simulink model "atrias_boom_nmSt_kinSw_v3"  (R2015a)
settings: Solver=ode23t  StartTime=0.0  StopTime=t_end  FixedStep=0.001  MaxStep=1e-3  RelTol=1e-3
InitFcn:
  | addpath('../common/')
  | colors
StartFcn:
  | tic
StopFcn:
  | %stopscript
values from neighbouring files (symbols this model uses):
  dt_a_dTrunk_boom = 5    [main_1_nmSt_kinSw.m]    (also in main_2_nmSt_kinSw_v2.m; main_3_nmSt_kinSw_v3.m; main_4_nmSt_kinSw_v4.m)
  dt_fade_boomCtrl = 2    [main_1_nmSt_kinSw.m]    (also in main_2_nmSt_kinSw_v2.m; main_3_nmSt_kinSw_v3.m; main_4_nmSt_kinSw_v4.m)
  initial_boom_yaw = 15*pi/180    (= 0.261799387799)    [main_2_nmSt_kinSw_v2.m]    (also in main_3_nmSt_kinSw_v3.m; main_4_nmSt_kinSw_v4.m)
  kd_boom_roll_Ctrl = 0    [main_1_nmSt_kinSw - Copy.m]    (also in main_1_nmSt_kinSw.m; main_2_nmSt_kinSw_v2.m; main_3_nmSt_kinSw_v3.m; main_4_nmSt_kinSw_v4.m)
  kd_boom_yaw_Ctrl = 0.1*kp_boom_yaw_Ctrl    (= 100000000)    [main_1_nmSt_kinSw - Copy.m]    (also in main_1_nmSt_kinSw.m = 1000000000; main_2_nmSt_kinSw_v2.m = 10000000; main_3_nmSt_kinSw_v3.m = 10000000; main_4_nmSt_kinSw_v4.m = 10000000)
  kd_motor = 0.90*2*sqrt(3.75*kp_motor)    [main_1_nmSt_kinSw - Copy.m]
  kinSw_alpha_start = 100*pi/180    (= 1.74532925199)    [main_1_nmSt_kinSw - Copy.m]    (also in main_1_nmSt_kinSw.m = 1.91986217719; main_2_nmSt_kinSw_v2.m = 1.83259571459; main_3_nmSt_kinSw_v3.m = 1.83259571459; main_4_nmSt_kinSw_v4.m = 1.83259571459)
  kinSw_alpha_tgt = 80*pi/180    (= 1.3962634016)    [main_1_nmSt_kinSw - Copy.m]    (also in main_1_nmSt_kinSw.m = 1.2217304764; main_2_nmSt_kinSw_v2.m = 1.2217304764; main_3_nmSt_kinSw_v3.m = 1.2217304764; main_4_nmSt_kinSw_v4.m = 1.2217304764)
  kinSw_t_start = 1.5    [main_1_nmSt_kinSw - Copy.m]    (also in main_1_nmSt_kinSw.m; main_2_nmSt_kinSw_v2.m = 0.5; main_3_nmSt_kinSw_v3.m = 0.5; main_4_nmSt_kinSw_v4.m = 0.5)
  kp_boom_roll_Ctrl = 0    [main_1_nmSt_kinSw - Copy.m]    (also in main_1_nmSt_kinSw.m; main_2_nmSt_kinSw_v2.m; main_3_nmSt_kinSw_v3.m; main_4_nmSt_kinSw_v4.m)
  kp_boom_yaw_Ctrl = 1e9    (= 1000000000)    [main_1_nmSt_kinSw - Copy.m]    (also in main_1_nmSt_kinSw.m = 10000000000; main_2_nmSt_kinSw_v2.m = 100000000; main_3_nmSt_kinSw_v3.m = 100000000; main_4_nmSt_kinSw_v4.m = 100000000)
  kp_motor = 3000    [main_1_nmSt_kinSw - Copy.m]
  max_back_bar_angle = 262.4*pi/180    (= 4.57974395723)    [main_1_nmSt_kinSw - Copy.m]
  max_front_bar_angle = 194.8*pi/180    (= 3.39990138288)    [main_1_nmSt_kinSw - Copy.m]
  min_back_bar_angle = 165.0*pi/180    (= 2.87979326579)    [main_1_nmSt_kinSw - Copy.m]
  min_front_bar_angle = 98.0*pi/180    (= 1.71042266695)    [main_1_nmSt_kinSw - Copy.m]
  poser_LLegAlp = (initial_l_leg_angle -pi/2)*180/pi    (= 105)    [main_2_nmSt_kinSw_v2.m]    (also in main_3_nmSt_kinSw_v3.m; main_4_nmSt_kinSw_v4.m)
  poser_LLegLen = initial_l_leg_length    (= 0.88)    [main_2_nmSt_kinSw_v2.m]    (also in main_3_nmSt_kinSw_v3.m; main_4_nmSt_kinSw_v4.m)
  poser_RLegAlp = (initial_r_leg_angle -pi/2)*180/pi    (= 75)    [main_2_nmSt_kinSw_v2.m]    (also in main_3_nmSt_kinSw_v3.m; main_4_nmSt_kinSw_v4.m)
  poser_RLegLen = initial_r_leg_length    (= 0.9)    [main_2_nmSt_kinSw_v2.m]    (also in main_3_nmSt_kinSw_v3.m; main_4_nmSt_kinSw_v4.m)
  tEnd_boomCtrl = t_end    (= 20)    [main_1_nmSt_kinSw - Copy.m]    (also in main_1_nmSt_kinSw.m = 3; main_2_nmSt_kinSw_v2.m = 7.5; main_3_nmSt_kinSw_v3.m = 7.5; main_4_nmSt_kinSw_v4.m = 7.5)
  tStart_boomCtrl = 1    [main_1_nmSt_kinSw - Copy.m]    (also in main_1_nmSt_kinSw.m = 0; main_2_nmSt_kinSw_v2.m = 0.5; main_3_nmSt_kinSw_v3.m = 0.5; main_4_nmSt_kinSw_v4.m = 0.5)
  tune_kinSw_alpha_start = kinSw_alpha_start*180/pi    (= 105)    [main_2_nmSt_kinSw_v2.m]    (also in main_3_nmSt_kinSw_v3.m; main_4_nmSt_kinSw_v4.m)
  tune_kinSw_alpha_tgt = kinSw_alpha_tgt*180/pi    (= 70)    [main_2_nmSt_kinSw_v2.m]    (also in main_3_nmSt_kinSw_v3.m; main_4_nmSt_kinSw_v4.m)
  tune_kinSw_len_min = kinSw_lclr    (= 0.7)    [main_2_nmSt_kinSw_v2.m]    (also in main_3_nmSt_kinSw_v3.m = 0.6)
  tune_kinSw_len_tgt = kinSw_len_tgt    (= 0.9)    [main_2_nmSt_kinSw_v2.m]    (also in main_3_nmSt_kinSw_v3.m)
  tune_M1_G = St_FGain_VAS*FmaxVAS    [main_2_nmSt_kinSw_v2.m]    (also in main_3_nmSt_kinSw_v3.m; main_4_nmSt_kinSw_v4.m)
  tune_M3_0 = CtrlPar_theta0*180/pi    [main_2_nmSt_kinSw_v2.m]    (also in main_3_nmSt_kinSw_v3.m; main_4_nmSt_kinSw_v4.m)
  tune_M3_D = St_GainDTh_HFL    [main_2_nmSt_kinSw_v2.m]    (also in main_3_nmSt_kinSw_v3.m; main_4_nmSt_kinSw_v4.m)
  tune_M3_P = St_GainTh_HFL    [main_2_nmSt_kinSw_v2.m]    (also in main_3_nmSt_kinSw_v3.m; main_4_nmSt_kinSw_v4.m)
  tune_M4_G = 1    [main_3_nmSt_kinSw_v3.m]    (also in main_4_nmSt_kinSw_v4.m)
  v_dTrunk_boom = 1.3    [main_1_nmSt_kinSw.m]    (also in main_2_nmSt_kinSw_v2.m; main_3_nmSt_kinSw_v3.m; main_4_nmSt_kinSw_v4.m)
undefined symbols (not defined in the file or in its folder): A1_notch_f1, A2_notch_f1, A_lpf_dtau, A_lpf_velocity, ankle_stiffness, B1_lpf_dtau, B1_lpf_velocity, B1_notch_f1, B2_lpf_dtau, B2_lpf_velocity, B2_notch_f1, b_hmotor, b_leg_spring, b_rotor, base_color_d, boom_color_d, boom_mount_to_center_diagonal, breakaway_friction, c_jointstop, contactThr, coulomb_friction, d_com, delta_phi_max, delta_phi_max_buffer, delta_phi_max_dropoff, delta_phi_min, fblink_color_d, floor_color_d, FmaxBFSH, FmaxGLU, FmaxHAM, FmaxHFL, FmaxRF, FmaxVAS, foot_color_d, FPCtrlPar, friction_linear_zone, g, gain_nodes_sea_torque, HIP_MTR_MAX_CONT_TORQUE, HIP_MTR_MAX_TORQUE, hshaft_color_d, initial_boom_pitch, initial_boom_roll, initial_hip_roll, initial_winch_angle, j_motor, k_gn, k_gt, k_leg_spring, K_notch_f1, k_phi, k_sea, Kb_leg, kd_lateral, kd_shin_max, kd_shin_min, kd_splay_max, kd_splay_min, kd_thigh_max ... (+186)
libraries: sm_lib x210, nesl_utility x140, simulink x65, simulink_extras x32, fl_lib x16, mblibv1 x2, commnoisgen2 x1
(part 10 of 17)

== system atrias_boom_nmSt_kinSw_v3/Mechanical System Layer/R Leg/Mechanical Limits/Shin Max Collision Model ==
  note: Mechanical Limits Model
  phi [rad] : Inport
  vphi [rad/s] : Inport  Port=2
  Contact! : EnablePort  StatesWhenEnabling=reset
  Gain3 : Gain  Gain=k_phi
  Gain4 : Gain  Gain=1/v_phi_max
  Mux1 : Mux  Inputs=2
  Reaction Force : Fcn  Expr="- u(1)  *  (1-u(2)) * (u(2)<1)"
  tau_interaction[Nm] : Outport  OutputWhenDisabled=reset  InitialOutput=0
      settings: AttributesFormatString=initial = '%<InitialOutput>'\nwhen disabled = '%<OutputWhenDisabled>'
  wires:
  Gain4/1 -> Mux1/2
  Gain3/1 -> Mux1/1
  Mux1/1 -> Reaction Force/1
  vphi [rad/s]/1 -> Gain4/1
  phi [rad]/1 -> Gain3/1
  Reaction Force/1 -> tau_interaction[Nm]/1

== system atrias_boom_nmSt_kinSw_v3/Mechanical System Layer/R Leg/Mechanical Limits/Shin Min Collision Model ==
  note: Mechanical Limits Model
  phi [rad] : Inport
  vphi [rad/s] : Inport  Port=2
  Contact! : EnablePort  StatesWhenEnabling=reset
  Gain3 : Gain  Gain=k_phi
  Gain4 : Gain  Gain=1/v_phi_max
  Mux1 : Mux  Inputs=2
  Reaction Force : Fcn  Expr="- u(1)  *  (1-u(2)) * (u(2)<1)"
  tau_interaction[Nm] : Outport  OutputWhenDisabled=reset  InitialOutput=0
      settings: AttributesFormatString=initial = '%<InitialOutput>'\nwhen disabled = '%<OutputWhenDisabled>'
  wires:
  Gain4/1 -> Mux1/2
  Gain3/1 -> Mux1/1
  Mux1/1 -> Reaction Force/1
  vphi [rad/s]/1 -> Gain4/1
  phi [rad]/1 -> Gain3/1
  Reaction Force/1 -> tau_interaction[Nm]/1

== system atrias_boom_nmSt_kinSw_v3/Mechanical System Layer/R Leg/Mechanical Limits/Thigh Max Collision Model ==
  note: Mechanical Limits Model
  phi [rad] : Inport
  vphi [rad/s] : Inport  Port=2
  Contact! : EnablePort  StatesWhenEnabling=reset
  Gain3 : Gain  Gain=k_phi
  Gain4 : Gain  Gain=1/v_phi_max
  Mux1 : Mux  Inputs=2
  Reaction Force : Fcn  Expr="- u(1)  *  (1-u(2)) * (u(2)<1)"
  tau_interaction[Nm] : Outport  OutputWhenDisabled=reset  InitialOutput=0
      settings: AttributesFormatString=initial = '%<InitialOutput>'\nwhen disabled = '%<OutputWhenDisabled>'
  wires:
  Gain4/1 -> Mux1/2
  Gain3/1 -> Mux1/1
  Mux1/1 -> Reaction Force/1
  vphi [rad/s]/1 -> Gain4/1
  phi [rad]/1 -> Gain3/1
  Reaction Force/1 -> tau_interaction[Nm]/1

== system atrias_boom_nmSt_kinSw_v3/Mechanical System Layer/R Leg/Mechanical Limits/Thigh Min Collision Model ==
  note: Mechanical Limits Model
  phi [rad] : Inport
  vphi [rad/s] : Inport  Port=2
  Contact! : EnablePort  StatesWhenEnabling=reset
  Gain3 : Gain  Gain=k_phi
  Gain4 : Gain  Gain=1/v_phi_max
  Mux1 : Mux  Inputs=2
  Reaction Force : Fcn  Expr="- u(1)  *  (1-u(2)) * (u(2)<1)"
  tau_interaction[Nm] : Outport  OutputWhenDisabled=reset  InitialOutput=0
      settings: AttributesFormatString=initial = '%<InitialOutput>'\nwhen disabled = '%<OutputWhenDisabled>'
  wires:
  Reaction Force/1 -> tau_interaction[Nm]/1
  phi [rad]/1 -> Gain3/1
  vphi [rad/s]/1 -> Gain4/1
  Mux1/1 -> Reaction Force/1
  Gain3/1 -> Mux1/1
  Gain4/1 -> Mux1/2

== system atrias_boom_nmSt_kinSw_v3/Mechanical System Layer/R Leg/Mechanical Limits/Thigh-Shin Collision Model ==
  note: Mechanical Limits Model
  delta_phi [rad] : Inport
  vphi [rad/s] : Inport  Port=2
  Contact! : EnablePort  StatesWhenEnabling=reset
  Gain3 : Gain  Gain=k_phi
  Gain4 : Gain  Gain=1/v_phi_max
  Mux1 : Mux  Inputs=2
  Reaction Force : Fcn  Expr="- u(1)  *  (1-u(2)) * (u(2)<1)"
  tau_interaction[Nm] : Outport  OutputWhenDisabled=reset  InitialOutput=0
      settings: AttributesFormatString=initial = '%<InitialOutput>'\nwhen disabled = '%<OutputWhenDisabled>'
  wires:
  Reaction Force/1 -> tau_interaction[Nm]/1
  delta_phi [rad]/1 -> Gain3/1
  vphi [rad/s]/1 -> Gain4/1
  Mux1/1 -> Reaction Force/1
  Gain3/1 -> Mux1/1
  Gain4/1 -> Mux1/2

== system atrias_boom_nmSt_kinSw_v3/Mechanical System Layer/R Leg/Mechanical Limits/Thigh-Shin Collision Model1 ==
  note: Mechanical Limits Model
  delta_phi [rad] : Inport
  vphi [rad/s] : Inport  Port=2
  Contact! : EnablePort  StatesWhenEnabling=reset
  Gain3 : Gain  Gain=k_phi
  Gain4 : Gain  Gain=1/v_phi_max
  Mux1 : Mux  Inputs=2
  Reaction Force : Fcn  Expr="- u(1)  *  (1-u(2)) * (u(2)<1)"
  tau_interaction[Nm] : Outport  OutputWhenDisabled=reset  InitialOutput=0
      settings: AttributesFormatString=initial = '%<InitialOutput>'\nwhen disabled = '%<OutputWhenDisabled>'
  wires:
  Reaction Force/1 -> tau_interaction[Nm]/1
  delta_phi [rad]/1 -> Gain3/1
  vphi [rad/s]/1 -> Gain4/1
  Mux1/1 -> Reaction Force/1
  Gain3/1 -> Mux1/1
  Gain4/1 -> Mux1/2

== system atrias_boom_nmSt_kinSw_v3/Mechanical System Layer/R Leg/Shin/Frame Data ==
  Kinematic Data : ToWorkspace  VariableName=r_shin_out  SampleTime=output_sample_time
      settings: Save2DSignal=2-D array (concatenate along first dimension)
  Mux : Mux
  PS-Simulink Converter{,1..3} (4 alike) : nesl_utility/PS-Simulink Converter  PhysicalDomain=network_engine_domain  SubClassName=ps_output  LeftPortType=input  RightPortType=output  PseudoPeriodic=off  Frequencies=[]  Unit=1  AffineConversion=off
  Transform Sensor : sm_lib/Frames and Transforms/Transform Sensor  MeasurementFrame=World  SenseAngle=off  SenseAxis=off  SenseAngle1=off  SenseAngle2=off  SenseAngle3=off  SenseQ=on  SenseR=off  SenseOmegaX=off  SenseOmegaY=off  SenseOmegaZ=off  SenseOmega1=off  SenseOmega2=off  SenseOmega3=off  SenseQDot=off  SenseRDot=off  SenseAlphaX=off  SenseAlphaY=off  SenseAlphaZ=off  SenseAlpha1=off  SenseAlpha2=off  SenseAlpha3=off  SenseQDDot=off  SenseRDDot=off  SenseX=on  SenseY=on  SenseZ=on  SenseRad=off  SenseAzim=off  SenseDist=off  SenseInc=off  SenseXDot=off  SenseYDot=off  SenseZDot=off  SenseRadDot=off  SenseAzimDot=off  SenseDistDot=off  SenseIncDot=off  SenseXDDot=off  SenseYDDot=off  SenseZDDot=off  SenseRadDDot=off  SenseAzimDDot=off  SenseDistDDot=off  SenseIncDDot=off  BlockFunction=simmechanics.library.frames_transforms.transform_sensor
  World Frame : sm_lib/Frames and Transforms/World Frame  BlockFunction=simmechanics.library.frames_transforms.world_frame
  Frame : PMIOPort  Port=1  Side=Left
  wires:
  Mux/1 -> Kinematic Data/1
  PS-Simulink Converter/1 -> Mux/1
  PS-Simulink Converter1/1 -> Mux/2
  PS-Simulink Converter2/1 -> Mux/3
  PS-Simulink Converter3/1 -> Mux/4
  connections:
  PS-Simulink Converter3/LConn1 -- Transform Sensor/RConn5
  PS-Simulink Converter2/LConn1 -- Transform Sensor/RConn4
  PS-Simulink Converter1/LConn1 -- Transform Sensor/RConn3
  PS-Simulink Converter/LConn1 -- Transform Sensor/RConn2
  Transform Sensor/RConn1 -- Frame/RConn1
  Transform Sensor/LConn1 -- World Frame/RConn1

== system atrias_boom_nmSt_kinSw_v3/Mechanical System Layer/R Leg/Shin SEA/Motor Controller ==
  Desired Current [A] : Inport
  Measured Current [A] : Inport  Port=2
  Speed [rad/s] : Inport  Port=3
  Ke : Gain  Gain=Kb_leg
  PI Controller : simulink/Continuous/PID Controller  Controller=PI  TimeDomain=Continuous-time  SampleTime=-1  IntegratorMethod=Trapezoidal  FilterMethod=Forward Euler  Form=Parallel  UseFilter=on  ControllerParametersSource=internal  P=0.57  I=0.016  D=0.016  N=10  InitialConditionSource=internal  InitialConditionForIntegrator=0  InitialConditionForFilter=0  ExternalReset=none  ZeroCross=off  LimitOutput=off  UpperSaturationLimit=inf  LowerSaturationLimit=-inf  LinearizeAsGain=on  AntiWindupMode=none  Kb=1  TrackingMode=off  Kt=1  PParamMin=[]  PParamMax=[]  IParamMin=[]  IParamMax=[]  DParamMin=[]  DParamMax=[]  NParamMin=[]  NParamMax=[]  KbParamMin=[]  KbParamMax=[]  KtParamMin=[]  KtParamMax=[]  POutMin=[]  POutMax=[]  IOutMin=[]  IOutMax=[]  DOutMin=[]  DOutMax=[]  NOutMin=[]  NOutMax=[]  KbOutMin=[]  KbOutMax=[]  KtOutMin=[]  KtOutMax=[]  IntegratorOutMin=[]  IntegratorOutMax=[]  FilterOutMin=[]  FilterOutMax=[]  SumOutMin=[]  SumOutMax=[]  SumI1OutMin=[]  SumI1OutMax=[]  SumI2OutMin=[]  SumI2OutMax=[]  SumI3OutMin=[]  SumI3OutMax=[]  SumDOutMin=[]  SumDOutMax=[]  SaturationOutMin=[]  SaturationOutMax=[]  IntegratorContinuousStateAttributes=''  IntegratorStateMustResolveToSignalObject=off  IntegratorRTWStateStorageClass=Auto  FilterContinuousStateAttributes=''  FilterStateMustResolveToSignalObject=off  FilterRTWStateStorageClass=Auto  DifferentiatorICPrevScaledInput=0  DifferentiatorOutMin=[]  DifferentiatorOutMax=[]
  Resistance : Gain  Gain=R_leg
  Sum : Sum  Inputs=|+-
  Sum1 : Sum  Inputs=|++
  Sum2 : Sum  Inputs=+|+
  Voltage [V] : Outport
  wires:
  Desired Current [A]/1 -> Sum/1
  Measured Current [A]/1 -> Resistance/1, Sum/2
  Sum/1 -> PI Controller/1
  PI Controller/1 -> Sum1/1
  Speed [rad/s]/1 -> Ke/1
  Sum2/1 -> Sum1/2
  Resistance/1 -> Sum2/1
  Ke/1 -> Sum2/2
  Sum1/1 -> Voltage [V]/1

== system atrias_boom_nmSt_kinSw_v3/Mechanical System Layer/R Leg/Shin SEA/Motor Electromagnetism ==
  Voltage [V] : Inport
  Speed [rad/s] : Inport  Port=2
  Add : Sum  Inputs=-+-
  Inductance : Gain  Gain=1/L_leg
  Integrator : Integrator  ZeroCross=off
  Ke : Gain  Gain=Kb_leg
  Resistance : Gain  Gain=R_leg
  Torque Limiter (outside) 1 : Saturate  UpperLimit=max_voltage_leg  LowerLimit=-max_voltage_leg  ZeroCross=off
      settings: AttributesFormatString=Hi: %<UpperLimit>\nLo: %<LowerLimit>
  Torque Limiter (outside) 2 : Saturate  UpperLimit=max_current_leg  LowerLimit=-max_current_leg  ZeroCross=off
      settings: AttributesFormatString=Hi: %<UpperLimit>\nLo: %<LowerLimit>
  Current [A] : Outport
  wires:
  Integrator/1 -> Torque Limiter (outside) 2/1  "I"
  Inductance/1 -> Integrator/1  "d/dt(I)"
  Speed [rad/s]/1 -> Ke/1  "d/dt(theta)"
  Add/1 -> Inductance/1
  Resistance/1 -> Add/1
  Ke/1 -> Add/3
  Voltage [V]/1 -> Torque Limiter (outside) 1/1
  Torque Limiter (outside) 1/1 -> Add/2
  Torque Limiter (outside) 2/1 -> Resistance/1, Current [A]/1

== system atrias_boom_nmSt_kinSw_v3/Mechanical System Layer/R Leg/Shin SEA/Rotor and Gearing ==
  Rotor Torque [Nm] : Inport
  Spring Torque [Nm] : Inport  Port=2
  Aligned Gear Constraint : sm_lib/Gears and Couplings/Gears/Common Gear Constraint  GearType=External  SpecificationType=CenterDistanceRatio  CenterDistance=(r_rotor+r_virtual_gear)/2  CenterDistanceUnits=m  GearRatio=1  BaseGearRadius=1  BaseGearRadiusUnits=m  FollGearRadius=1  FollGearRadiusUnits=m  AssemblyGearRotation=Free  BlockFunction=simmechanics.library.gears_couplings_drives.gears.common_gear
  External Force and Torque : sm_lib/Forces and Torques/External Force and Torque  ForceResolutionFrame=AttachedFrame  EnableForceX=off  EnableForceY=off  EnableForceZ=off  EnableForce=off  TorqueResolutionFrame=AttachedFrame  EnableTorqueX=off  EnableTorqueY=off  EnableTorqueZ=on  EnableTorque=off  BlockFunction=simmechanics.library.forces_torques.external_force_torque
  Gear Offset : sm_lib/Frames and Transforms/Rigid Transform  TranslationMethod=Cartesian  TranslationLengthUnit=m  TranslationStandardAxis=+Z  TranslationStandardOffset=0  TranslationCartesianOffset=[(r_rotor+r_virtual_gear) 0 0]  TranslationROffset=0  TranslationROffsetUnits=m  TranslationZOffset=0  TranslationZOffsetUnits=m  TranslationThetaOffset=0  TranslationThetaOffsetUnits=deg  RotationMethod=None  RotationAngleUnits=deg  RotationStandardAxis=+Z  RotationAngle=0  RotationArbitraryAxis=[0 0 1]  FollAlignAxisA=+X  BaseAlignAxisA=+Y  FollAlignAxisB=+Y  BaseAlignAxisB=+Z  RotationMatrix=[1 0 0; 0 1 0; 0 0 1]  BlockFunction=simmechanics.library.frames_transforms.rigid_transform
  Idler Gear : sm_lib/Body Elements/Solid  InertiaType=Custom  Mass=m_virtual_gear  MassUnits=kg  CenterOfMass=[0 0 0]  CenterOfMassUnits=m  MomentsOfInertia=i_virtual_gear  MomentsOfInertiaUnits=kg*m^2  ProductsOfInertia=[0 0 0]  ProductsOfInertiaUnits=kg*m^2  DensityBased=on  Density=1000  DensityUnits=kg/(m^3)  GraphicType=None  MarkerShape=Sphere  MarkerSize=10  MarkerSizeUnits=m  GraphicVisPropType=SimpleVisualProperties  GraphicDiffuseColor=[1.0 0.2 0.2]  GraphicSpecularColor=[0.5 0.5 0.5 1.0]  GraphicAmbientColor=[0.15 0.15 0.15 1.0]  GraphicEmissiveColor=[0.0 0.0 0.0 1.0]  GraphicShininess=75  GraphicOpacity=1.0  GeometryShape=Cylinder  RectangleSize=[1 1]  RectangleSizeUnits=m  BrickDimensions=[1 1 1]  BrickDimensionUnits=m  CylinderRadius=r_virtual_gear  CylinderRadiusUnits=m  CylinderLength=0.01  CylinderLengthUnits=m  SphereRadius=1  SphereRadiusUnits=m  EllipsoidRadii=[1 1 1]  EllipsoidRadiiUnits=m  ExtrusionCrossSection=[1 1; -1 1; -1 -1; 1 -1]  ExtrusionCrossSectionUnits=m  ExtrusionLength=.2  ExtrusionLengthUnits=m  PolygonNumSides=3  PolygonOuterRadius=.3  PolygonOuterRadiusUnits=m  ExtGeomFileType=STL  ExtGeomFileUnits=m  RevolutionCrossSection=[1 1; 1 -1; 2 -1; 2 1]  RevolutionCrossSectionUnits=m  RevolutionExtent=Full  RevolutionAngle=180  RevolutionAngleUnits=deg  BlockFunction=simmechanics.library.body_elements.solid
  Idler Gear Constraint : sm_lib/Gears and Couplings/Gears/Common Gear Constraint  GearType=External  SpecificationType=CenterDistanceRatio  CenterDistance=(r_rotor+r_virtual_gear)/2  CenterDistanceUnits=m  GearRatio=1.0  BaseGearRadius=r_rotor  BaseGearRadiusUnits=m  FollGearRadius=r_virtual_gear  FollGearRadiusUnits=m  AssemblyGearRotation=Free  BlockFunction=simmechanics.library.gears_couplings_drives.gears.common_gear
  Idler Offset : sm_lib/Frames and Transforms/Rigid Transform  TranslationMethod=Cartesian  TranslationLengthUnit=m  TranslationStandardAxis=+Z  TranslationStandardOffset=0  TranslationCartesianOffset=[(r_rotor+r_virtual_gear)/2 0 0]  TranslationROffset=0  TranslationROffsetUnits=m  TranslationZOffset=0  TranslationZOffsetUnits=m  TranslationThetaOffset=0  TranslationThetaOffsetUnits=deg  RotationMethod=None  RotationAngleUnits=deg  RotationStandardAxis=+Z  RotationAngle=0  RotationArbitraryAxis=[0 0 1]  FollAlignAxisA=+X  BaseAlignAxisA=+Y  FollAlignAxisB=+Y  BaseAlignAxisB=+Z  RotationMatrix=[1 0 0; 0 1 0; 0 0 1]  BlockFunction=simmechanics.library.frames_transforms.rigid_transform
  Mechanical Rotational Reference : fl_lib/Mechanical/Rotational Elements/Mechanical Rotational Reference
  Opposite : Gain  Gain=-1
  Output Gear Joint : sm_lib/Joints/Revolute Joint  SenseConstraintForce=off  SenseConstraintForceX=off  SenseConstraintForceY=off  SenseConstraintForceZ=off  SenseConstraintTorque=off  SenseConstraintTorqueX=off  SenseConstraintTorqueY=off  SenseConstraintTorqueZ=off  SenseTotalForce=off  SenseTotalForceX=off  SenseTotalForceY=off  SenseTotalForceZ=off  SenseTotalTorque=off  SenseTotalTorqueX=off  SenseTotalTorqueY=off  SenseTotalTorqueZ=off  CompositeWrenchDir=FollowerOnBase  CompositeWrenchFrame=BaseFrame  EquilibriumPosition=0  EquilibriumPositionUnits=deg  SpringStiffness=0  SpringStiffnessUnits=N*m/deg  DampingCoefficient=0  DampingCoefficientUnits=N*m/(deg/s)  TorqueActuationMode=NoTorque  MotionActuationMode=ComputedMotion  SensePosition=on  SenseVelocity=on  SenseAcceleration=off  SenseTorqueForce=off  PositionTargetSpecify=off  PositionTargetPriority=High  PositionTargetValue=0  PositionTargetValueUnits=deg  VelocityTargetSpecify=off  VelocityTargetPriority=High  VelocityTargetValue=0  VelocityTargetValueUnits=deg/s  BlockFunction=simmechanics.library.joints.revolute_joint
  Output Gear : sm_lib/Body Elements/Solid  InertiaType=Custom  Mass=m_output_gear  MassUnits=kg  CenterOfMass=[0 0 0]  CenterOfMassUnits=m  MomentsOfInertia=i_output_gear  MomentsOfInertiaUnits=kg*m^2  ProductsOfInertia=[0 0 0]  ProductsOfInertiaUnits=kg*m^2  DensityBased=on  Density=1000  DensityUnits=kg/(m^3)  GraphicType=None  MarkerShape=Sphere  MarkerSize=10  MarkerSizeUnits=m  GraphicVisPropType=SimpleVisualProperties  GraphicDiffuseColor=[1.0 0.2 0.0]  GraphicSpecularColor=[0.5 0.5 0.5 1.0]  GraphicAmbientColor=[0.15 0.15 0.15 1.0]  GraphicEmissiveColor=[0.0 0.0 0.0 1.0]  GraphicShininess=75  GraphicOpacity=1.0  GeometryShape=Cylinder  RectangleSize=[1 1]  RectangleSizeUnits=m  BrickDimensions=[1 1 1]  BrickDimensionUnits=m  CylinderRadius=0.03  CylinderRadiusUnits=m  CylinderLength=0.01  CylinderLengthUnits=m  SphereRadius=1  SphereRadiusUnits=m  EllipsoidRadii=[1 1 1]  EllipsoidRadiiUnits=m  ExtrusionCrossSection=[1 1; -1 1; -1 -1; 1 -1]  ExtrusionCrossSectionUnits=m  ExtrusionLength=1  ExtrusionLengthUnits=m  PolygonNumSides=3  PolygonOuterRadius=1  PolygonOuterRadiusUnits=m  ExtGeomFileType=STL  ExtGeomFileUnits=m  RevolutionCrossSection=[1 1; 1 -1; 2 -1; 2 1]  RevolutionCrossSectionUnits=m  RevolutionExtent=Full  RevolutionAngle=180  RevolutionAngleUnits=deg  BlockFunction=simmechanics.library.body_elements.solid
  PS-Simulink Converter{,1..3} (4 alike) : nesl_utility/PS-Simulink Converter  PhysicalDomain=network_engine_domain  SubClassName=ps_output  LeftPortType=input  RightPortType=output  PseudoPeriodic=off  Frequencies=[]  Unit=1  AffineConversion=off
  Rotational Simscape Intf : Subsystem
  Rotational Friction : fl_lib/Mechanical/Rotational Elements/Rotational Friction  brkwy_trq=breakaway_friction(1)/N N*m  Col_trq=coulomb_friction(1)/N N*m  visc_coef=viscous_friction(1)/N N*m/(rad/s)  trans_coef=10 s/rad  vel_thr=friction_linear_zone(1)*N rad/s  w_specify=off  w_priority=High  w=0 rad/s  t_specify=off  t_priority=High  t=0 N*m
  Rotor + Base Gear : sm_lib/Body Elements/Solid  InertiaType=Custom  Mass=m_rotor  MassUnits=kg  CenterOfMass=[0 0 0]  CenterOfMassUnits=m  MomentsOfInertia=i_rotor_moments  MomentsOfInertiaUnits=kg*m^2  ProductsOfInertia=[0 0 0]  ProductsOfInertiaUnits=kg*m^2  DensityBased=on  Density=1000  DensityUnits=kg/(m^3)  GraphicType=None  MarkerShape=Sphere  MarkerSize=10  MarkerSizeUnits=m  GraphicVisPropType=AdvancedVisualProperties  GraphicDiffuseColor=[0.5 0.5 0.5]  GraphicSpecularColor=[0.5 0.5 0.5 1.0]  GraphicAmbientColor=[0.15 0.15 0.15 1.0]  GraphicEmissiveColor=[0.0 0.0 0.0 1.0]  GraphicShininess=10  GraphicOpacity=1.0  GeometryShape=Cylinder  RectangleSize=[1 1]  RectangleSizeUnits=m  BrickDimensions=[1 1 1]  BrickDimensionUnits=m  CylinderRadius=0.01  CylinderRadiusUnits=m  CylinderLength=0.01  CylinderLengthUnits=m  SphereRadius=1  SphereRadiusUnits=m  EllipsoidRadii=[1 1 1]  EllipsoidRadiiUnits=m  ExtrusionCrossSection=[1 1; -1 1; -1 -1; 1 -1]  ExtrusionCrossSectionUnits=m  ExtrusionLength=0.4  ExtrusionLengthUnits=m  PolygonNumSides=3  PolygonOuterRadius=0.2  PolygonOuterRadiusUnits=m  ExtGeomFileType=STL  ExtGeomFileUnits=m  RevolutionCrossSection=[1 1; 1 -1; 2 -1; 2 1]  RevolutionCrossSectionUnits=m  RevolutionExtent=Full  RevolutionAngle=180  RevolutionAngleUnits=deg  BlockFunction=simmechanics.library.body_elements.solid
  Rotor Joint : sm_lib/Joints/Revolute Joint  SenseConstraintForce=off  SenseConstraintForceX=off  SenseConstraintForceY=off  SenseConstraintForceZ=off  SenseConstraintTorque=off  SenseConstraintTorqueX=off  SenseConstraintTorqueY=off  SenseConstraintTorqueZ=off  SenseTotalForce=off  SenseTotalForceX=off  SenseTotalForceY=off  SenseTotalForceZ=off  SenseTotalTorque=off  SenseTotalTorqueX=off  SenseTotalTorqueY=off  SenseTotalTorqueZ=off  CompositeWrenchDir=FollowerOnBase  CompositeWrenchFrame=BaseFrame  EquilibriumPosition=0  EquilibriumPositionUnits=deg  SpringStiffness=0  SpringStiffnessUnits=N*m/deg  DampingCoefficient=0  DampingCoefficientUnits=N*m/(deg/s)  TorqueActuationMode=InputTorque  MotionActuationMode=ComputedMotion  SensePosition=off  SenseVelocity=on  SenseAcceleration=off  SenseTorqueForce=off  PositionTargetSpecify=off  PositionTargetPriority=High  PositionTargetValue=0  PositionTargetValueUnits=deg  VelocityTargetSpecify=off  VelocityTargetPriority=High  VelocityTargetValue=0  VelocityTargetValueUnits=deg/s  BlockFunction=simmechanics.library.joints.revolute_joint
  Simulink-PS Converter : nesl_utility/Simulink-PS Converter  PhysicalDomain=network_engine_domain  SubClassName=ps_input  LeftPortType=input  RightPortType=output  PseudoPeriodic=off  Frequencies=[]  NoiseDistribution=none  NoiseParameters=[]  Unit=1  AffineConversion=off  InputFiltering=off  SimscapeFilterOrder=1  InputFilterTimeConstant=0.001  UdotUserProvided=1
  Simulink-PS Converter1 : nesl_utility/Simulink-PS Converter  PhysicalDomain=network_engine_domain  SubClassName=ps_input  LeftPortType=input  RightPortType=output  PseudoPeriodic=off  Frequencies=[]  NoiseDistribution=none  NoiseParameters=[]  Unit=1  AffineConversion=off  InputFiltering=off  SimscapeFilterOrder=1  InputFilterTimeConstant=0.001  UdotUserProvided=1
  Sum : Sum  Inputs=|++
  Virtual Gear Joint : sm_lib/Joints/Revolute Joint  SenseConstraintForce=off  SenseConstraintForceX=off  SenseConstraintForceY=off  SenseConstraintForceZ=off  SenseConstraintTorque=off  SenseConstraintTorqueX=off  SenseConstraintTorqueY=off  SenseConstraintTorqueZ=off  SenseTotalForce=off  SenseTotalForceX=off  SenseTotalForceY=off  SenseTotalForceZ=off  SenseTotalTorque=off  SenseTotalTorqueX=off  SenseTotalTorqueY=off  SenseTotalTorqueZ=off  CompositeWrenchDir=FollowerOnBase  CompositeWrenchFrame=BaseFrame  EquilibriumPosition=0  EquilibriumPositionUnits=deg  SpringStiffness=0  SpringStiffnessUnits=N*m/deg  DampingCoefficient=0  DampingCoefficientUnits=N*m/(deg/s)  TorqueActuationMode=NoTorque  MotionActuationMode=ComputedMotion  SensePosition=off  SenseVelocity=off  SenseAcceleration=off  SenseTorqueForce=off  PositionTargetSpecify=off  PositionTargetPriority=High  PositionTargetValue=0  PositionTargetValueUnits=deg  VelocityTargetSpecify=off  VelocityTargetPriority=High  VelocityTargetValue=0  VelocityTargetValueUnits=deg/s  BlockFunction=simmechanics.library.joints.revolute_joint
  Virtual Follower Gear : sm_lib/Body Elements/Solid  InertiaType=Custom  Mass=m_virtual_gear  MassUnits=kg  CenterOfMass=[0 0 0]  CenterOfMassUnits=m  MomentsOfInertia=i_virtual_gear  MomentsOfInertiaUnits=kg*m^2  ProductsOfInertia=[0 0 0]  ProductsOfInertiaUnits=kg*m^2  DensityBased=on  Density=1000  DensityUnits=kg/(m^3)  GraphicType=None  MarkerShape=Sphere  MarkerSize=10  MarkerSizeUnits=m  GraphicVisPropType=SimpleVisualProperties  GraphicDiffuseColor=[1.0 0.2 0.2]  GraphicSpecularColor=[0.5 0.5 0.5 1.0]  GraphicAmbientColor=[0.15 0.15 0.15 1.0]  GraphicEmissiveColor=[0.0 0.0 0.0 1.0]  GraphicShininess=75  GraphicOpacity=1.0  GeometryShape=Cylinder  RectangleSize=[1 1]  RectangleSizeUnits=m  BrickDimensions=[1 1 1]  BrickDimensionUnits=m  CylinderRadius=r_virtual_gear  CylinderRadiusUnits=m  CylinderLength=0.01  CylinderLengthUnits=m  SphereRadius=1  SphereRadiusUnits=m  EllipsoidRadii=[1 1 1]  EllipsoidRadiiUnits=m  ExtrusionCrossSection=[1 1; -1 1; -1 -1; 1 -1]  ExtrusionCrossSectionUnits=m  ExtrusionLength=.2  ExtrusionLengthUnits=m  PolygonNumSides=3  PolygonOuterRadius=.3  PolygonOuterRadiusUnits=m  ExtGeomFileType=STL  ExtGeomFileUnits=m  RevolutionCrossSection=[1 1; 1 -1; 2 -1; 2 1]  RevolutionCrossSectionUnits=m  RevolutionExtent=Full  RevolutionAngle=180  RevolutionAngleUnits=deg  BlockFunction=simmechanics.library.body_elements.solid
  Virtual Gear Constraint : sm_lib/Gears and Couplings/Gears/Common Gear Constraint  GearType=External  SpecificationType=PitchCircleRadii  CenterDistance=20.0  CenterDistanceUnits=cm  GearRatio=1.0  BaseGearRadius=r_rotor  BaseGearRadiusUnits=m  FollGearRadius=r_virtual_gear  FollGearRadiusUnits=m  AssemblyGearRotation=Free  BlockFunction=simmechanics.library.gears_couplings_drives.gears.common_gear
  Virtual Idler : sm_lib/Joints/Revolute Joint  SenseConstraintForce=off  SenseConstraintForceX=off  SenseConstraintForceY=off  SenseConstraintForceZ=off  SenseConstraintTorque=off  SenseConstraintTorqueX=off  SenseConstraintTorqueY=off  SenseConstraintTorqueZ=off  SenseTotalForce=off  SenseTotalForceX=off  SenseTotalForceY=off  SenseTotalForceZ=off  SenseTotalTorque=off  SenseTotalTorqueX=off  SenseTotalTorqueY=off  SenseTotalTorqueZ=off  CompositeWrenchDir=FollowerOnBase  CompositeWrenchFrame=BaseFrame  EquilibriumPosition=0  EquilibriumPositionUnits=deg  SpringStiffness=0  SpringStiffnessUnits=N*m/deg  DampingCoefficient=0  DampingCoefficientUnits=N*m/(deg/s)  TorqueActuationMode=NoTorque  MotionActuationMode=ComputedMotion  SensePosition=off  SenseVelocity=off  SenseAcceleration=off  SenseTorqueForce=off  PositionTargetSpecify=off  PositionTargetPriority=High  PositionTargetValue=0  PositionTargetValueUnits=deg  VelocityTargetSpecify=off  VelocityTargetPriority=High  VelocityTargetValue=0  VelocityTargetValueUnits=deg/s  BlockFunction=simmechanics.library.joints.revolute_joint
  Rotor Conn : PMIOPort  Port=1  Side=Left
  Gearhead Position [rad] : Outport
  Gearhead Velocity [rad/s] : Outport  Port=2
  Rotor Velocity [rad/s] : Outport  Port=3
  wires:
  PS-Simulink Converter1/1 -> Gearhead Position [rad]/1
  Rotor Torque [Nm]/1 -> Sum/1
  PS-Simulink Converter2/1 -> Gearhead Velocity [rad/s]/1
  PS-Simulink Converter3/1 -> Rotor Velocity [rad/s]/1
  Spring Torque [Nm]/1 -> Opposite/1
  Opposite/1 -> Simulink-PS Converter1/1
  PS-Simulink Converter/1 -> Sum/2
  Sum/1 -> Simulink-PS Converter/1
  connections:
  Virtual Gear Joint/RConn1 -- Virtual Follower Gear/RConn1 -- Virtual Gear Constraint/RConn1 -- Idler Gear Constraint/LConn1
  External Force and Torque/RConn1 -- Output Gear/RConn1 -- Aligned Gear Constraint/RConn1 -- Output Gear Joint/RConn1
  Gear Offset/RConn1 -- Virtual Gear Joint/LConn1
  Gear Offset/LConn1 -- Rotor Joint/LConn1 -- Rotor Conn/RConn1 -- Output Gear Joint/LConn1 -- Idler Offset/LConn1
  Rotor Joint/RConn1 -- Virtual Gear Constraint/LConn1 -- Rotor + Base Gear/RConn1
  Rotor Joint/LConn2 -- Simulink-PS Converter/RConn1
  PS-Simulink Converter2/LConn1 -- Output Gear Joint/RConn3
  PS-Simulink Converter1/LConn1 -- Output Gear Joint/RConn2
  PS-Simulink Converter3/LConn1 -- Rotational Simscape Intf/LConn1 -- Rotor Joint/RConn2
  Simulink-PS Converter1/RConn1 -- External Force and Torque/LConn1
  Idler Gear Constraint/RConn1 -- Virtual Idler/RConn1 -- Idler Gear/RConn1 -- Aligned Gear Constraint/LConn1
  Idler Offset/RConn1 -- Virtual Idler/LConn1
  Rotational Simscape Intf/RConn2 -- Mechanical Rotational Reference/LConn1 -- Rotational Friction/RConn1
  Rotational Friction/LConn1 -- Rotational Simscape Intf/LConn2
  PS-Simulink Converter/LConn1 -- Rotational Simscape Intf/RConn1

== system atrias_boom_nmSt_kinSw_v3/Mechanical System Layer/R Leg/Thigh/Frame Data ==
  Kinematic Data : ToWorkspace  VariableName=r_thigh_out  SampleTime=output_sample_time
      settings: Save2DSignal=2-D array (concatenate along first dimension)
  Mux : Mux
  PS-Simulink Converter{,1..3} (4 alike) : nesl_utility/PS-Simulink Converter  PhysicalDomain=network_engine_domain  SubClassName=ps_output  LeftPortType=input  RightPortType=output  PseudoPeriodic=off  Frequencies=[]  Unit=1  AffineConversion=off
  Transform Sensor : sm_lib/Frames and Transforms/Transform Sensor  MeasurementFrame=World  SenseAngle=off  SenseAxis=off  SenseAngle1=off  SenseAngle2=off  SenseAngle3=off  SenseQ=on  SenseR=off  SenseOmegaX=off  SenseOmegaY=off  SenseOmegaZ=off  SenseOmega1=off  SenseOmega2=off  SenseOmega3=off  SenseQDot=off  SenseRDot=off  SenseAlphaX=off  SenseAlphaY=off  SenseAlphaZ=off  SenseAlpha1=off  SenseAlpha2=off  SenseAlpha3=off  SenseQDDot=off  SenseRDDot=off  SenseX=on  SenseY=on  SenseZ=on  SenseRad=off  SenseAzim=off  SenseDist=off  SenseInc=off  SenseXDot=off  SenseYDot=off  SenseZDot=off  SenseRadDot=off  SenseAzimDot=off  SenseDistDot=off  SenseIncDot=off  SenseXDDot=off  SenseYDDot=off  SenseZDDot=off  SenseRadDDot=off  SenseAzimDDot=off  SenseDistDDot=off  SenseIncDDot=off  BlockFunction=simmechanics.library.frames_transforms.transform_sensor
  World Frame : sm_lib/Frames and Transforms/World Frame  BlockFunction=simmechanics.library.frames_transforms.world_frame
  Frame : PMIOPort  Port=1  Side=Left
  wires:
  Mux/1 -> Kinematic Data/1
  PS-Simulink Converter/1 -> Mux/1
  PS-Simulink Converter1/1 -> Mux/2
  PS-Simulink Converter2/1 -> Mux/3
  PS-Simulink Converter3/1 -> Mux/4
  connections:
  PS-Simulink Converter3/LConn1 -- Transform Sensor/RConn5
  PS-Simulink Converter2/LConn1 -- Transform Sensor/RConn4
  PS-Simulink Converter1/LConn1 -- Transform Sensor/RConn3
  PS-Simulink Converter/LConn1 -- Transform Sensor/RConn2
  Transform Sensor/RConn1 -- Frame/RConn1
  Transform Sensor/LConn1 -- World Frame/RConn1

== system atrias_boom_nmSt_kinSw_v3/Mechanical System Layer/R Leg/Thigh SEA/Motor Controller ==
  Desired Current [A] : Inport
  Measured Current [A] : Inport  Port=2
  Speed [rad/s] : Inport  Port=3
  Ke : Gain  Gain=Kb_leg
  PI Controller : simulink/Continuous/PID Controller  Controller=PI  TimeDomain=Continuous-time  SampleTime=-1  IntegratorMethod=Trapezoidal  FilterMethod=Forward Euler  Form=Parallel  UseFilter=on  ControllerParametersSource=internal  P=0.57  I=0.016  D=0.016  N=10  InitialConditionSource=internal  InitialConditionForIntegrator=0  InitialConditionForFilter=0  ExternalReset=none  ZeroCross=off  LimitOutput=off  UpperSaturationLimit=inf  LowerSaturationLimit=-inf  LinearizeAsGain=on  AntiWindupMode=none  Kb=1  TrackingMode=off  Kt=1  PParamMin=[]  PParamMax=[]  IParamMin=[]  IParamMax=[]  DParamMin=[]  DParamMax=[]  NParamMin=[]  NParamMax=[]  KbParamMin=[]  KbParamMax=[]  KtParamMin=[]  KtParamMax=[]  POutMin=[]  POutMax=[]  IOutMin=[]  IOutMax=[]  DOutMin=[]  DOutMax=[]  NOutMin=[]  NOutMax=[]  KbOutMin=[]  KbOutMax=[]  KtOutMin=[]  KtOutMax=[]  IntegratorOutMin=[]  IntegratorOutMax=[]  FilterOutMin=[]  FilterOutMax=[]  SumOutMin=[]  SumOutMax=[]  SumI1OutMin=[]  SumI1OutMax=[]  SumI2OutMin=[]  SumI2OutMax=[]  SumI3OutMin=[]  SumI3OutMax=[]  SumDOutMin=[]  SumDOutMax=[]  SaturationOutMin=[]  SaturationOutMax=[]  IntegratorContinuousStateAttributes=''  IntegratorStateMustResolveToSignalObject=off  IntegratorRTWStateStorageClass=Auto  FilterContinuousStateAttributes=''  FilterStateMustResolveToSignalObject=off  FilterRTWStateStorageClass=Auto  DifferentiatorICPrevScaledInput=0  DifferentiatorOutMin=[]  DifferentiatorOutMax=[]
  Resistance : Gain  Gain=R_leg
  Sum : Sum  Inputs=|+-
  Sum1 : Sum  Inputs=|++
  Sum2 : Sum  Inputs=+|+
  Voltage [V] : Outport
  wires:
  Desired Current [A]/1 -> Sum/1
  Measured Current [A]/1 -> Resistance/1, Sum/2
  Sum/1 -> PI Controller/1
  PI Controller/1 -> Sum1/1
  Speed [rad/s]/1 -> Ke/1
  Sum2/1 -> Sum1/2
  Resistance/1 -> Sum2/1
  Ke/1 -> Sum2/2
  Sum1/1 -> Voltage [V]/1

== system atrias_boom_nmSt_kinSw_v3/Mechanical System Layer/R Leg/Thigh SEA/Motor Electromagnetism ==
  Voltage [V] : Inport
  Speed [rad/s] : Inport  Port=2
  Add : Sum  Inputs=-+-
  Inductance : Gain  Gain=1/L_leg
  Integrator : Integrator  ZeroCross=off
  Ke : Gain  Gain=Kb_leg
  Resistance : Gain  Gain=R_leg
  Torque Limiter (outside) 1 : Saturate  UpperLimit=max_voltage_leg  LowerLimit=-max_voltage_leg  ZeroCross=off
      settings: AttributesFormatString=Hi: %<UpperLimit>\nLo: %<LowerLimit>
  Torque Limiter (outside) 2 : Saturate  UpperLimit=max_current_leg  LowerLimit=-max_current_leg  ZeroCross=off
      settings: AttributesFormatString=Hi: %<UpperLimit>\nLo: %<LowerLimit>
  Current [A] : Outport
  wires:
  Integrator/1 -> Torque Limiter (outside) 2/1  "I"
  Inductance/1 -> Integrator/1  "d/dt(I)"
  Speed [rad/s]/1 -> Ke/1  "d/dt(theta)"
  Add/1 -> Inductance/1
  Resistance/1 -> Add/1
  Ke/1 -> Add/3
  Voltage [V]/1 -> Torque Limiter (outside) 1/1
  Torque Limiter (outside) 2/1 -> Current [A]/1, Resistance/1
  Torque Limiter (outside) 1/1 -> Add/2
